simulink model "Discrete_observer"  (R2021b)
settings: Solver=VariableStepAuto  StartTime=0.0  StopTime=10.0  RelTol=1e-3
values from neighbouring files (symbols this model uses):
  A1 = expm(A(2:4,2:4)*0.01)    [simulation_models.m]
  B1 = (A1-eye(3))*inv(A(2:4,2:4))*B(2:4)    [simulation_models.m]
  L1 = L1'    [simulation_models.m]
  M = 22.304    [parameters.m]    (also in simulation_models.m)
undefined symbols (not defined in the file or in its folder): DiscIntNeverNeededParam
settings Model: Creator=szmis  LastModifiedBy=szmis

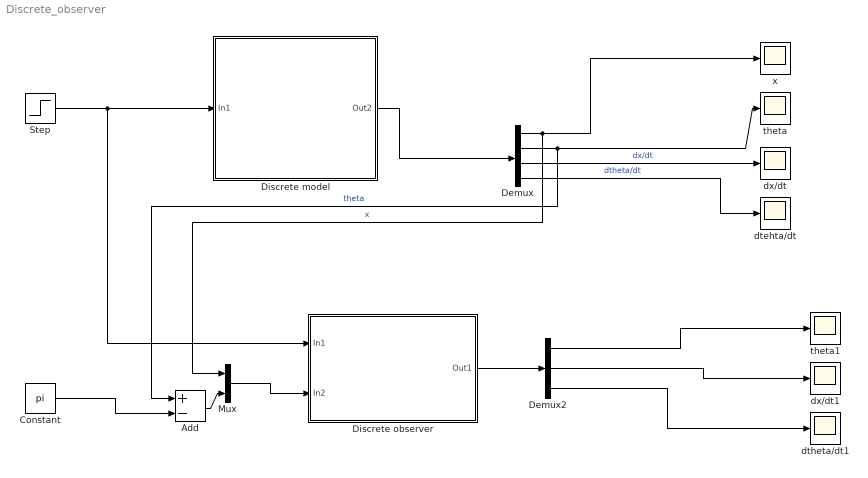
== system Discrete_observer ==
  Add : Sum  Inputs=+-
  Constant : Constant  Value=pi
  Demux : Demux
  Demux2 : Demux  Outputs=3
  Discrete model : Subsystem
  Discrete observer : Subsystem
  Mux : Mux  Inputs=2
  Step : Step  After=0.3  SampleTime=0
  dtehta/dt : Scope
  dtheta/dt1 : Scope
  dx/dt : Scope
  dx/dt1 : Scope
  theta : Scope
  theta1 : Scope
  x : Scope
  wires:
  Discrete observer/1(Out1) -> Demux2/1
  Demux2/3 -> dtheta/dt1/1
  Demux/2 -> theta/1, Add/1  "theta"
  Step/1 -> Discrete model/1(In1), Discrete observer/1(In1)
  Demux/4 -> dtehta/dt/1  "dtheta/dt"
  Demux/3 -> dx/dt/1  "dx/dt"
  Demux2/1 -> theta1/1
  Discrete model/1(Out2) -> Demux/1
  Constant/1 -> Add/2
  Add/1 -> Mux/2
  Demux2/2 -> dx/dt1/1
  Demux/1 -> Mux/1, x/1  "x"
  Mux/1 -> Discrete observer/2(In2)

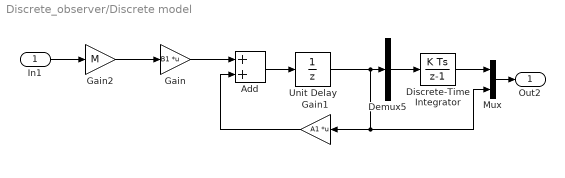
== system Discrete_observer/Discrete model ==
  In1 : Inport
  Add : Sum
  Demux5 : Demux  Outputs=3
  Discrete-Time Integrator : DiscreteIntegrator  SampleTime=0.1  ICPrevOutput=DiscIntNeverNeededParam  ICPrevScaledInput=DiscIntNeverNeededParam
  Gain : Gain  Gain=B1  Multiplication=Matrix(K*u)  SampleTime=0.1
  Gain1 : Gain  Gain=A1  Multiplication=Matrix(K*u)  SampleTime=0.1
  Gain2 : Gain  Gain=M  SampleTime=0.1
  Mux : Mux  Inputs=2
  Unit Delay : UnitDelay  SampleTime=0.1  HasFrameUpgradeWarning=on
  Out2 : Outport
  wires:
  Add/1 -> Unit Delay/1
  Gain/1 -> Add/1
  Gain1/1 -> Add/2
  Unit Delay/1 -> Demux5/1, Gain1/1, Mux/2
  Gain2/1 -> Gain/1
  Discrete-Time Integrator/1 -> Mux/1
  Demux5/2 -> Discrete-Time Integrator/1
  In1/1 -> Gain2/1
  Mux/1 -> Out2/1

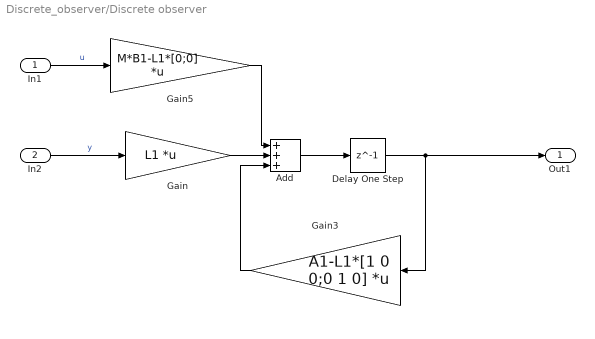
== system Discrete_observer/Discrete observer ==
  In1 : Inport
  In2 : Inport  Port=2
  Add : Sum  Inputs=+++
  Delay One Step : Delay  DelayLength=1
  Gain : Gain  Gain=L1  Multiplication=Matrix(K*u)
  Gain3 : Gain  Gain=A1-L1*[1 0 0;0 1 0]  Multiplication=Matrix(K*u)
  Gain5 : Gain  Gain=M*B1-L1*[0;0]  Multiplication=Matrix(K*u)
  Out1 : Outport
  wires:
  In2/1 -> Gain/1  "y"
  Delay One Step/1 -> Gain3/1, Out1/1
  Add/1 -> Delay One Step/1
  In1/1 -> Gain5/1  "u"
  Gain/1 -> Add/2
  Gain3/1 -> Add/3
  Gain5/1 -> Add/1
